simulink model "nilib"  (Simulink 6.2)
settings: Solver=ode45  SolverMode=SingleTasking  StartTime=0.0  StopTime=999999  MaxStep=10  RelTol=1e-3  AbsTol=1e-3
settings Model: Creator=jacobs  LastModifiedBy=jacobs  ExtModeAutoUpdateStatusClock=off
settings DataIOCC: LimitDataPoints=off  SaveOutput=off  SaveTime=off
settings OptimizationCC: BlockReduction=off  BooleanDataType=off
settings HardwareCC: TargetUnknown=on
settings STFCustomTargetCC: TargetFcnLib=ansi_tfl_tmw.mat  GenFloatMathFcnCalls=ANSI_C  ModelReferenceCompliant=off  SystemTargetFile=grt.tlc

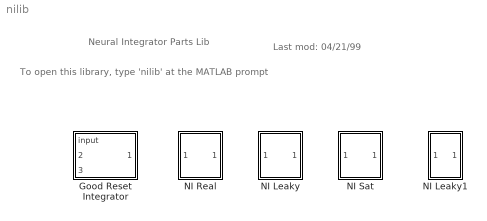
== system nilib ==
  note: Neural Integrator Parts Lib
  note: To open this library, type 'nilib'
      | at the MATLAB prompt
  note: Last mod:
      | 04/21/99
  Good Reset Integrator : Subsystem
      mask Display: disp('Resettable\nNI')
  NI Leaky : Subsystem
      mask Display: disp('NI\nLeaky')
  NI Leaky1 : Subsystem
      mask Display: disp('N\nLeaky')
  NI Real : Subsystem
      mask Display: disp('NI\nReal')
  NI Sat : Subsystem
      mask Display: disp('NI\nSat')

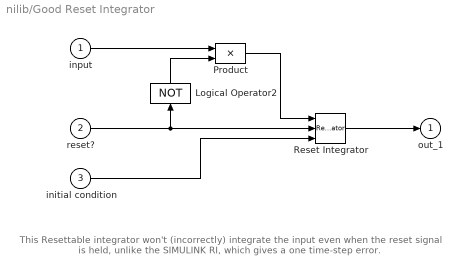
== system nilib/Good Reset Integrator ==
  note: This Resettable integrator won't (incorrectly) integrate the input even
      | when the reset signal is held, unlike the SIMULINK RI, which
      | gives a one time-step error.
  input : Inport  Port=1  LatchInput=off
  reset? : Inport  Port=2  LatchInput=off
  initial condition : Inport  Port=3  LatchInput=off
  Logical Operator2 : Logic  Orientation=up  Operator=NOT  Inputs=1
  Product : Product  SaturateOnIntegerOverflow=on  RndMeth=Zero  InputSameDT=on
  Reset Integrator : ResetIntegrator
  out_1 : Outport  InitialOutput=0
  wires:
  reset?/1 -> Logical Operator2/1, Reset Integrator/2
  Product/1 -> Reset Integrator/1
  input/1 -> Product/1
  Logical Operator2/1 -> Product/2
  initial condition/1 -> Reset Integrator/3
  Reset Integrator/1 -> out_1/1

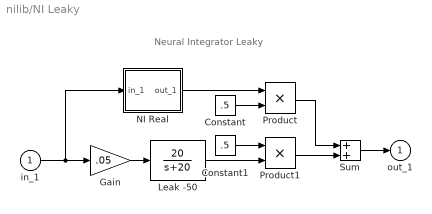
== system nilib/NI Leaky ==
  note: Neural Integrator Leaky
  in_1 : Inport  Port=1  LatchInput=off
  Constant : Constant  Value=.5
  Constant1 : Constant  Value=.5
  Gain : Gain  Gain=.05  SaturateOnIntegerOverflow=on
  Leak -50 : TransferFcn  Numerator=20  Denominator=[1 20]
  NI Real : Subsystem
      mask Display: disp('NI Real')
  Product : Product  SaturateOnIntegerOverflow=on  RndMeth=Zero  InputSameDT=on
  Product1 : Product  SaturateOnIntegerOverflow=on  RndMeth=Zero  InputSameDT=on
  Sum : Sum  SaturateOnIntegerOverflow=on  InputSameDT=on
  out_1 : Outport  InitialOutput=0
  wires:
  Sum/1 -> out_1/1
  Product1/1 -> Sum/2
  Gain/1 -> Leak -50/1
  in_1/1 -> Gain/1, NI Real/1(in_1)
  Leak -50/1 -> Product1/2
  Constant1/1 -> Product1/1
  Product/1 -> Sum/1
  NI Real/1(out_1) -> Product/1
  Constant/1 -> Product/2

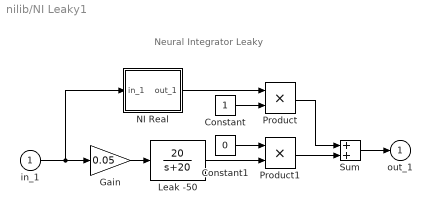
== system nilib/NI Leaky1 ==
  note: Neural Integrator Leaky
  in_1 : Inport  Port=1  LatchInput=off
  Constant : Constant
  Constant1 : Constant  Value=0
  Gain : Gain  Gain=0.05  SaturateOnIntegerOverflow=on
  Leak -50 : TransferFcn  Numerator=20  Denominator=[1 20]
  NI Real : Subsystem
      mask Display: disp('NI Real')
  Product : Product  SaturateOnIntegerOverflow=on  RndMeth=Zero  InputSameDT=on
  Product1 : Product  SaturateOnIntegerOverflow=on  RndMeth=Zero  InputSameDT=on
  Sum : Sum  SaturateOnIntegerOverflow=on  InputSameDT=on
  out_1 : Outport  InitialOutput=0
  wires:
  Constant/1 -> Product/2
  NI Real/1(out_1) -> Product/1
  Product/1 -> Sum/1
  Constant1/1 -> Product1/1
  Leak -50/1 -> Product1/2
  in_1/1 -> NI Real/1(in_1), Gain/1
  Gain/1 -> Leak -50/1
  Product1/1 -> Sum/2
  Sum/1 -> out_1/1

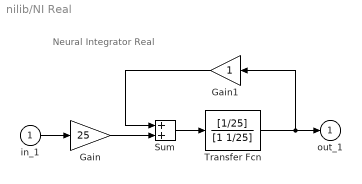
== system nilib/NI Real ==
  note: Neural Integrator Real
  in_1 : Inport  Port=1  LatchInput=off
  Gain : Gain  Gain=25  SaturateOnIntegerOverflow=on
  Gain1 : Gain  Orientation=left  SaturateOnIntegerOverflow=on
  Sum : Sum  SaturateOnIntegerOverflow=on  InputSameDT=on
  Transfer Fcn : TransferFcn  Numerator=[1/25]  Denominator=[1 1/25]
  out_1 : Outport  InitialOutput=0
  wires:
  in_1/1 -> Gain/1
  Gain/1 -> Sum/2
  Sum/1 -> Transfer Fcn/1
  Gain1/1 -> Sum/1
  Transfer Fcn/1 -> out_1/1, Gain1/1

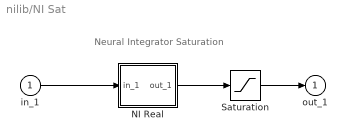
== system nilib/NI Sat ==
  note: Neural Integrator Saturation
  in_1 : Inport  Port=1  LatchInput=off
  NI Real : Subsystem
      mask Display: disp('NI Real')
  Saturation : Saturate  UpperLimit=20  LowerLimit=-20
  out_1 : Outport  InitialOutput=0
  wires:
  in_1/1 -> NI Real/1(in_1)
  Saturation/1 -> out_1/1
  NI Real/1(out_1) -> Saturation/1

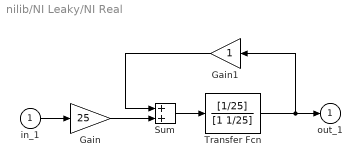
== system nilib/NI Leaky/NI Real ==
  in_1 : Inport  Port=1  LatchInput=off
  Gain : Gain  Gain=25  SaturateOnIntegerOverflow=on
  Gain1 : Gain  Orientation=left  SaturateOnIntegerOverflow=on
  Sum : Sum  SaturateOnIntegerOverflow=on  InputSameDT=on
  Transfer Fcn : TransferFcn  Numerator=[1/25]  Denominator=[1 1/25]
  out_1 : Outport  InitialOutput=0
  wires:
  Transfer Fcn/1 -> Gain1/1, out_1/1
  Gain1/1 -> Sum/1
  Sum/1 -> Transfer Fcn/1
  Gain/1 -> Sum/2
  in_1/1 -> Gain/1

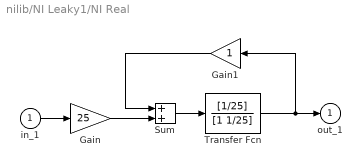
== system nilib/NI Leaky1/NI Real ==
  in_1 : Inport  Port=1  LatchInput=off
  Gain : Gain  Gain=25  SaturateOnIntegerOverflow=on
  Gain1 : Gain  Orientation=left  SaturateOnIntegerOverflow=on
  Sum : Sum  SaturateOnIntegerOverflow=on  InputSameDT=on
  Transfer Fcn : TransferFcn  Numerator=[1/25]  Denominator=[1 1/25]
  out_1 : Outport  InitialOutput=0
  wires:
  in_1/1 -> Gain/1
  Gain/1 -> Sum/2
  Sum/1 -> Transfer Fcn/1
  Gain1/1 -> Sum/1
  Transfer Fcn/1 -> out_1/1, Gain1/1

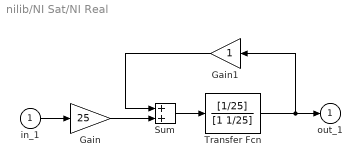
== system nilib/NI Sat/NI Real ==
  in_1 : Inport  Port=1  LatchInput=off
  Gain : Gain  Gain=25  SaturateOnIntegerOverflow=on
  Gain1 : Gain  Orientation=left  SaturateOnIntegerOverflow=on
  Sum : Sum  SaturateOnIntegerOverflow=on  InputSameDT=on
  Transfer Fcn : TransferFcn  Numerator=[1/25]  Denominator=[1 1/25]
  out_1 : Outport  InitialOutput=0
  wires:
  Transfer Fcn/1 -> Gain1/1, out_1/1
  Gain1/1 -> Sum/1
  Sum/1 -> Transfer Fcn/1
  Gain/1 -> Sum/2
  in_1/1 -> Gain/1
